simulink model "live_run"  (Simulink 6.6)
settings: Solver=ode45  StartTime=0.0  StopTime=5  RelTol=1e-3
values from neighbouring files (symbols this model uses):
  desired_states = [set_point.theta; set_point.omega]    [set_parameters.m]    (also in tablesat3.m = str2num(get(handles.set_points,'String')))
  PID = evalin('base','PID')    [tablesat3.m]
undefined symbols (not defined in the file or in its folder): flag
settings Model: Creator=Cooch  LastModifiedBy=Administrator
settings DebuggingCC: AlgebraicLoopMsg=none  SolverPrmCheckMsg=none  UnconnectedInputMsg=none  UnconnectedOutputMsg=none  UnconnectedLineMsg=none

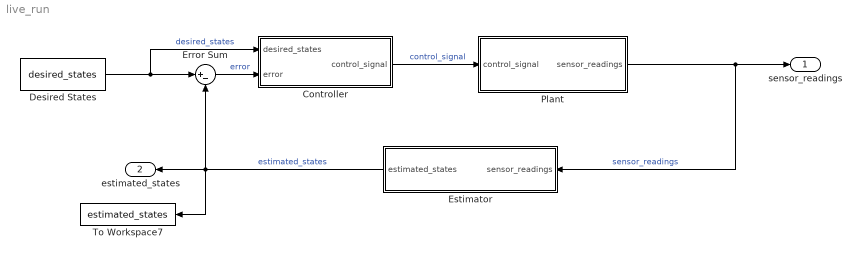
== system live_run ==
  Controller : Subsystem
  Desired States : Constant  Value=desired_states
  Error Sum : Sum  Inputs=|+-
  Estimator : Subsystem  Orientation=left
  Plant : Subsystem
  To Workspace7 : ToWorkspace  VariableName=estimated_states  SampleTime=-1  SaveFormat=Array
  sensor_readings : Outport
  estimated_states : Outport  Orientation=left  Port=2
  wires:
  Desired States/1 -> Error Sum/1, Controller/1(desired_states)  "desired_states"
  Error Sum/1 -> Controller/2(error)  "error"
  Controller/1(control_signal) -> Plant/1(control_signal)  "control_signal"
  Estimator/1(estimated_states) -> Error Sum/2, estimated_states/1, To Workspace7/1  "estimated_states"
  Plant/1(sensor_readings) -> Estimator/1(sensor_readings), sensor_readings/1  "sensor_readings"

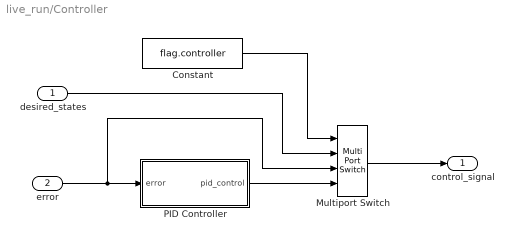
== system live_run/Controller ==
  desired_states : Inport
  error : Inport  Port=2
  Constant : Constant  Value=flag.controller
  Multiport Switch : MultiPortSwitch  Inputs=3  zeroidx=on
  PID Controller : Subsystem
  control_signal : Outport
  wires:
  error/1 -> Multiport Switch/3, PID Controller/1(error)
  Multiport Switch/1 -> control_signal/1
  Constant/1 -> Multiport Switch/1
  PID Controller/1(pid_control) -> Multiport Switch/4
  desired_states/1 -> Multiport Switch/2

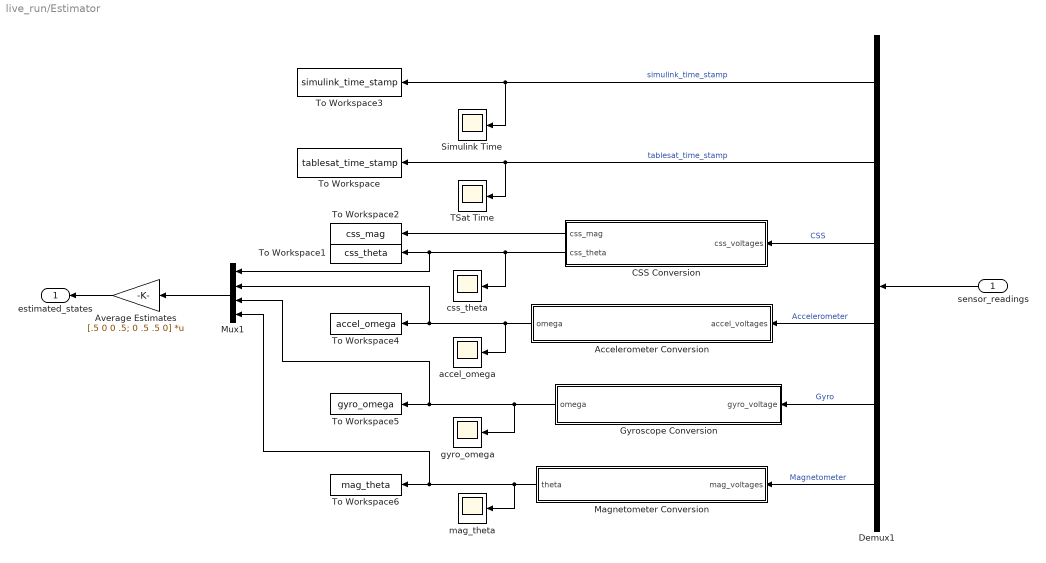
== system live_run/Estimator ==
  sensor_readings : Inport  Orientation=left
  Accelerometer Conversion : Stateflow chart  Orientation=left
  Average Estimates : Gain  Orientation=left  Gain=[.5 0 0 .5; 0 .5 .5 0]  Multiplication=Matrix(K*u)
  CSS Conversion : Stateflow chart  Orientation=left
  Demux1 : Demux  Orientation=left  Outputs=[1;1;6;4;1;3]
  Gyroscope Conversion : Stateflow chart  Orientation=left
  Magnetometer Conversion : Stateflow chart  Orientation=left
  Mux1 : Mux  Orientation=left
  Simulink Time : Scope
      settings: TimeRange=10  YMin=0  YMax=10
  TSat Time : Scope
      settings: SaveName=ScopeData2
  To Workspace : ToWorkspace  VariableName=tablesat_time_stamp  SampleTime=-1  SaveFormat=Array
  To Workspace1 : ToWorkspace  VariableName=css_theta  SampleTime=-1  SaveFormat=Array
  To Workspace2 : ToWorkspace  VariableName=css_mag  SampleTime=-1  SaveFormat=Array
  To Workspace3 : ToWorkspace  VariableName=simulink_time_stamp  SampleTime=-1  SaveFormat=Array
  To Workspace4 : ToWorkspace  VariableName=accel_omega  SampleTime=-1  SaveFormat=Array
  To Workspace5 : ToWorkspace  VariableName=gyro_omega  SampleTime=-1  SaveFormat=Array
  To Workspace6 : ToWorkspace  VariableName=mag_theta  SampleTime=-1  SaveFormat=Array
  accel_omega : Scope
      settings: YMin=2.5  YMax=4.25  SaveName=ScopeData3
  css_theta : Scope
  gyro_omega : Scope
      settings: SaveName=ScopeData4
  mag_theta : Scope
      settings: SaveName=ScopeData5
  estimated_states : Outport  Orientation=left
  wires:
  Demux1/1 -> Simulink Time/1, To Workspace3/1  "simulink_time_stamp"
  Demux1/2 -> TSat Time/1, To Workspace/1  "tablesat_time_stamp"
  Demux1/3 -> CSS Conversion/1(css_voltages)  "CSS"
  Demux1/4 -> Accelerometer Conversion/1(accel_voltages)  "Accelerometer"
  Demux1/5 -> Gyroscope Conversion/1(gyro_voltage)  "Gyro"
  Demux1/6 -> Magnetometer Conversion/1(mag_voltages)  "Magnetometer"
  CSS Conversion/1(css_mag) -> To Workspace2/1
  CSS Conversion/2(css_theta) -> css_theta/1, To Workspace1/1, Mux1/1
  Accelerometer Conversion/1(omega) -> accel_omega/1, To Workspace4/1, Mux1/2
  Gyroscope Conversion/1(omega) -> gyro_omega/1, To Workspace5/1, Mux1/3
  Magnetometer Conversion/1(theta) -> mag_theta/1, To Workspace6/1, Mux1/4
  sensor_readings/1 -> Demux1/1
  Average Estimates/1 -> estimated_states/1
  Mux1/1 -> Average Estimates/1

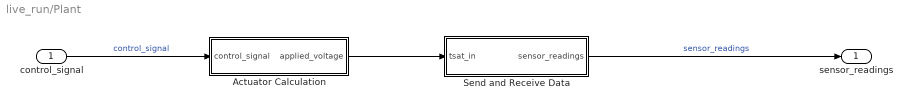
== system live_run/Plant ==
  control_signal : Inport
  Actuator Calculation : Subsystem
  Send and Receive Data : Subsystem
  sensor_readings : Outport
  wires:
  Actuator Calculation/1(applied_voltage) -> Send and Receive Data/1(tsat_in)
  control_signal/1 -> Actuator Calculation/1(control_signal)  "control_signal"
  Send and Receive Data/1(sensor_readings) -> sensor_readings/1  "sensor_readings"

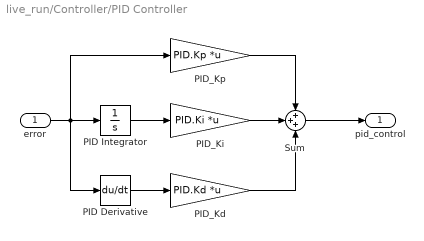
== system live_run/Controller/PID Controller ==
  error : Inport
  PID Derivative : Derivative
  PID Integrator : Integrator
  PID_Kd : Gain  Gain=PID.Kd  Multiplication=Matrix(K*u)
  PID_Ki : Gain  Gain=PID.Ki  Multiplication=Matrix(K*u)
  PID_Kp : Gain  Gain=PID.Kp  Multiplication=Matrix(K*u)
  Sum : Sum  Inputs=+++
  pid_control : Outport
  wires:
  PID Integrator/1 -> PID_Ki/1
  PID Derivative/1 -> PID_Kd/1
  PID_Kp/1 -> Sum/1
  error/1 -> PID_Kp/1, PID Integrator/1, PID Derivative/1
  PID_Ki/1 -> Sum/2
  PID_Kd/1 -> Sum/3
  Sum/1 -> pid_control/1

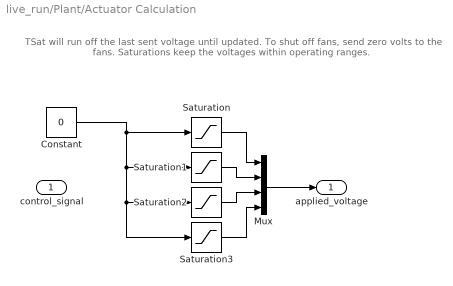
== system live_run/Plant/Actuator Calculation ==
  note: TSat will run off the last sent voltage until updated.
      | To shut off fans, send zero volts to the fans.
      |
      | Saturations keep the voltages within operating ranges.
  control_signal : Inport
  Constant : Constant  Value=0
  Mux : Mux
  Saturation{,1..3} (4 alike) : Saturate  UpperLimit=12  LowerLimit=0
  applied_voltage : Outport
  wires:
  Saturation/1 -> Mux/1
  Saturation1/1 -> Mux/2
  Saturation2/1 -> Mux/3
  Saturation3/1 -> Mux/4
  Mux/1 -> applied_voltage/1
  Constant/1 -> Saturation/1, Saturation1/1, Saturation2/1, Saturation3/1

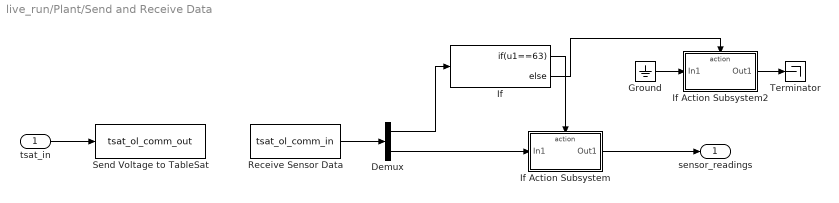
== system live_run/Plant/Send and Receive Data ==
  tsat_in : Inport
  Demux : Demux  Outputs=[1;-1]
  Ground : Ground
  If : If  IfExpression=u1==63
  If Action Subsystem : Subsystem  TreatAsAtomicUnit=on
  If Action Subsystem2 : Subsystem  TreatAsAtomicUnit=on
  Receive Sensor Data : S-Function  FunctionName=tsat_ol_comm_in
  Send Voltage to TableSat : S-Function  FunctionName=tsat_ol_comm_out
  Terminator : Terminator
  sensor_readings : Outport
  wires:
  tsat_in/1 -> Send Voltage to TableSat/1
  If/1 -> If Action Subsystem/Action
  If/2 -> If Action Subsystem2/Action
  Demux/1 -> If/1
  Receive Sensor Data/1 -> Demux/1
  If Action Subsystem2/1(Out1) -> Terminator/1
  Demux/2 -> If Action Subsystem/1(In1)
  Ground/1 -> If Action Subsystem2/1(In1)
  If Action Subsystem/1(Out1) -> sensor_readings/1

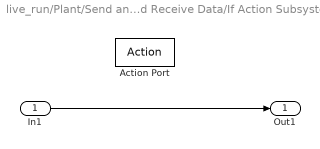
== system live_run/Plant/Send and Receive Data/If Action Subsystem ==
  In1 : Inport
  Action Port : ActionPort  ActionType=then
  Out1 : Outport
  wires:
  In1/1 -> Out1/1

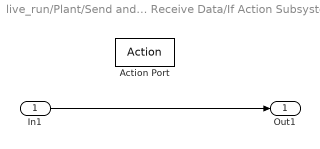
== system live_run/Plant/Send and Receive Data/If Action Subsystem2 ==
  In1 : Inport
  Action Port : ActionPort  ActionType=else
  Out1 : Outport
  wires:
  In1/1 -> Out1/1

== matlab function Estimator/Accelerometer Conversion ==
  data: accel_voltages input inherited; omega output inherited
function omega = accel_volt_to_omega( accel_voltages )
%ACCEL_VOLT_TO_OMEGA uses the two onboard dual axes accelerometers to
%determine the angular acceleration
%   Inputs:  vector of 4 accelerometer voltages.  Orientation is to be
%   determined.
%   
%   Output:  In first pass at sensor reading only return the rotation
%   about the major axis omega z.  Later development should determine
%   nutation about the x and y axes.
%
omega = 0;

== matlab function Estimator/CSS Conversion ==
  data: css_voltages input inherited; css_mag output inherited; css_theta output inherited
function [ css_mag, css_theta ] = css_to_theta( css_voltages )
%CSS_TO_THETA uses the six sun sensors to find the direction to the largest
%source of light.
%   Inputs:  vector of 6 css voltages.  CSS 1 is assumed to be zero
%   degrees.  An offset may be added to this code if a different zero is
%   needed.
%   
%   Outputs:  Using a resultant force style analysis.  The resultant
%   magnitude showing the strength of the signal and the resultant angle
%   theta are returned.
%
css_x=0;
css_y=0;
for n = 1:size(css_voltages,1)
    css_x = css_x + cos((n-1)*pi()/3)*css_voltages(n);
    css_y = css_y + sin((n-1)*pi()/3)*css_voltages(n);
end
css_mag = (css_x^2+css_y^2)^0.5;
css_theta = atan(css_y/css_x);
if css_x < o
    css_theta = css_theta+pi();
end
if css_theta < 0
    css_theta = css_theta + 2*pi();
end

== matlab function Estimator/Gyroscope Conversion ==
  data: gyro_voltage input inherited; omega output inherited
function omega = gyro_volt_to_omega( gyro_voltage )
%GYRO_VOLT_TO_OMEGA uses a single axis gyroscope to determine angular 
%rate of the tablesat.
%   Inputs:  single value of the gyroscope's voltage
%   
%   Output:  Calculated angular velocity.
%


%Missy used the following to convert gyro voltage to degrees per second.
%GyroValue = (cals->Volts2Dps * (GyroVolts - cals->GyroOffset));

omega = 0;

== matlab function Estimator/Magnetometer Conversion ==
  data: mag_voltages input inherited; theta output inherited
function theta = mag_volt_to_theta( mag_voltages )
%MAG_VOLT_TO_THETA uses the onboard 3-axes magnetometer to determine
%orientation.
%   Inputs:  vector of 3 magnetometer voltages.  Orientation is to be
%   determined.
%   
%   Output:  Orientation w.r.t. the vertical z-axis.
%
theta = 0;

%/* Calculate Unit Magnetic Vector (Bhat) */ 
%TamTemp[0] = cals->TamGain[0] * (MagXVolts - cals->TamBias[0]); 
%TamTemp[1] = cals->TamGain[1] * (MagYVolts - cals->TamBias[1]); 
%TamTemp[2] = cals->TamGain[2] * (MagZVolts - cals->TamBias[2]); 
%TamMag = sqrt(pow(TamTemp[0],2) + pow(TamTemp[1],2) + pow(TamTemp[2],2)); 
 
%BhatX = TamTemp[1]/TamMag; 
%BhatY = -TamTemp[0]/TamMag; 
%BhatZ = TamTemp[2]/TamMag; 
 
%/* Compute TAM azimuth */
%AzTam = -atan2(TamTemp[1],TamTemp[0])*Rad2Deg;
